simulink model "GolfSwingLogging"  (R2024b)
settings: Solver=VariableStepAuto  StartTime=0.0  StopTime=StopTime  MaxStep=0.001  RelTol=1e-3
PreLoadFcn:
  | cd(matlabdrive);
  | cd '2DModel';
PostLoadFcn:
  | %run SCRIPT_mdlWksGenerate.m;
  | mdlWks=get_param('GolfSwing','ModelWorkspace');
  | mdlWks.DataSource = 'MAT-File';
  | mdlWks.FileName = 'ModelInputs.mat';
  | mdlWks.reload;
model workspace: external: MAT-File ModelInputs.mat (data not in the file)
undefined symbols (not defined in the file or in its folder): GlobalGain, HipConstant, HipDampening, HipTimeGain, KillDampFinalValue, KillDampInitialValue, KillswitchFinalValue, KillswitchInitialValue, KillswitchStepTime, LElbowConstant, LElbowDampening, LElbowTimeGain, LScapConstant, LScapDampening, LScapPositionGain, LScapTimeGain, LShoulderConstant, LShoulderDampening, LShoulderTimeGain, LWristConstant, LWristDampening, LWristTimeGain, RElbowConstant, RElbowDampening, RElbowTimeGain, RScapConstant, RScapDampening, RScapPositionGain, RScapTimeGain, RShoulderConstant, RShoulderDampening, RShoulderTimeGain, RWristConstant, RWristDampening, RWristTimeGain, TorsoConstant, TorsoDampening, TorsoPositionGain, TorsoTimeGain, WristGain, X, Y, Z
libraries: nesl_utility x204, sm_lib x102, matrix_library x11, simulink_extras x2, simulink x1
(part 3 of 6)

== system GolfSwingLogging/Left Forearm MOF ==
  LW Global Position : Inport
  LE Global Position : Inport  Port=2
  LArmonLForearmFGlobalIn : Inport  Port=3
  LArmonLForearmTGlobalIn : Inport  Port=4
  LWristonLForearmFGlobalIn : Inport  Port=5
  LWristonLForearmTGlobalIn : Inport  Port=6
  LEAngularImpulseonForearm : Integrator
  LElbowonLForearmMOFGlobal : matrix_library/Cross Product
  LElbowonLForearmMOFLocal : Product  Multiplication=Matrix(*)
  LFCOM : sm_lib/Body Elements/Inertia Sensor  SensorExtent=BodyGroup  SpanWeldJoints=off  ExcludeGroundedBodies=off  MeasurementFrame=World  SenseMass=off  SenseCenterOfMass=on  SenseInertiaMatrix=off  SenseCenteredInertiaMatrix=off  SensePrincipalInertiaMatrix=off  SenseRotationMatrix=off  GraphicType=None  PrincipalInertiaFrameSize=20  GraphicVisPropType=SimpleVisualProperties  GraphicDiffuseColor=[0.5 0.5 0.5]  GraphicOpacity=1  GraphicSpecularColor=[0.5 0.5 0.5 1.0]  GraphicAmbientColor=[0.15 0.15 0.15 1.0]  GraphicEmissiveColor=[0.0 0.0 0.0 1.0]  GraphicShininess=75
  LWristonLForearmMOFGlobal : matrix_library/Cross Product
  LWristonLForearmMOFLocal : Product  Multiplication=Matrix(*)
  Left Forearm COM : nesl_utility/PS-Simulink Converter  PhysicalDomain=network_engine_domain  SubClassName=ps_output  LeftPortType=input  RightPortType=output  PseudoPeriodic=off  Frequencies=[]  VectorFormat=1-D array  Unit=inherit  AffineConversion=off
  R Vector Elbow Force on Left Forearm : Sum  Inputs=-+
  R Vector Wrist Force on Left Forearm : Sum  Inputs=-+
  RotationTransformLeftHand : nesl_utility/PS-Simulink Converter  PhysicalDomain=network_engine_domain  SubClassName=ps_output  LeftPortType=input  RightPortType=output  PseudoPeriodic=off  Frequencies=[]  VectorFormat=1-D array  Unit=inherit  AffineConversion=off
  SumofMomentsLEonLForearm : Sum
  SumofMomentsLForearmLocal : Product  Multiplication=Matrix(*)
  SumofMomentsLeftForearmGlobal : Sum  Inputs=++++
  Transform Sensor : sm_lib/Frames and Transforms/Transform Sensor  MeasurementFrame=World  RotationSequence=XYX  SenseAngle=off  SenseAxis=off  SenseQ=off  SenseR=on  SenseRotationSequence=off  SenseOmegaX=off  SenseOmegaY=off  SenseOmegaZ=off  SenseOmega=off  SenseQDot=off  SenseRDot=off  SenseRotationSequenceDot=off  SenseAlphaX=off  SenseAlphaY=off  SenseAlphaZ=off  SenseAlpha=off  SenseQDDot=off  SenseRDDot=off  SenseX=off  SenseY=off  SenseZ=off  SenseXYZ=off  SenseRad=off  SenseAzim=off  SenseDist=off  SenseInc=off  SenseXDot=off  SenseYDot=off  SenseZDot=off  SenseXYZDot=off  SenseRadDot=off  SenseAzimDot=off  SenseDistDot=off  SenseIncDot=off  SenseXDDot=off  SenseYDDot=off  SenseZDDot=off  SenseXYZDDot=off  SenseRadDDot=off  SenseAzimDDot=off  SenseDistDDot=off  SenseIncDDot=off
  World Frame : sm_lib/Frames and Transforms/World Frame
  Left Forearm : PMIOPort  Side=Left
  wires:
  Left Forearm COM/1 -> R Vector Elbow Force on Left Forearm/1, R Vector Wrist Force on Left Forearm/1  "LeftForearmCOM"
  LE Global Position/1 -> R Vector Elbow Force on Left Forearm/2
  LW Global Position/1 -> R Vector Wrist Force on Left Forearm/2
  R Vector Elbow Force on Left Forearm/1 -> LElbowonLForearmMOFGlobal/1
  LArmonLForearmFGlobalIn/1 -> LElbowonLForearmMOFGlobal/2
  R Vector Wrist Force on Left Forearm/1 -> LWristonLForearmMOFGlobal/1
  LWristonLForearmTGlobalIn/1 -> SumofMomentsLeftForearmGlobal/4
  LWristonLForearmFGlobalIn/1 -> LWristonLForearmMOFGlobal/2
  SumofMomentsLeftForearmGlobal/1 -> SumofMomentsLForearmLocal/2  "SumofMomentsLeftForearmGlobal"
  LWristonLForearmMOFGlobal/1 -> LWristonLForearmMOFLocal/2, SumofMomentsLeftForearmGlobal/2  "LWristonLForearmMOFGlobal"
  RotationTransformLeftHand/1 -> SumofMomentsLForearmLocal/1, LWristonLForearmMOFLocal/1, LElbowonLForearmMOFLocal/1
  LElbowonLForearmMOFGlobal/1 -> SumofMomentsLEonLForearm/2, LElbowonLForearmMOFLocal/2, SumofMomentsLeftForearmGlobal/1  "LElbowonLForearmMOFGlobal"
  SumofMomentsLEonLForearm/1 -> LEAngularImpulseonForearm/1  "SumofMomentsLEonLForearm"
  LArmonLForearmTGlobalIn/1 -> SumofMomentsLEonLForearm/1, SumofMomentsLeftForearmGlobal/3
  connections:
  LFCOM/LConn1 -- Transform Sensor/LConn1 -- Left Forearm/RConn1
  LFCOM/RConn1 -- Left Forearm COM/LConn1
  Transform Sensor/RConn1 -- World Frame/RConn1
  RotationTransformLeftHand/LConn1 -- Transform Sensor/RConn2

== system GolfSwingLogging/Left Scapula Joint ==
  note: LSOutput
  LScapForce : nesl_utility/PS-Simulink Converter  PhysicalDomain=network_engine_domain  SubClassName=ps_output  LeftPortType=input  RightPortType=output  PseudoPeriodic=off  Frequencies=[]  VectorFormat=1-D array  Unit=inherit  AffineConversion=off
  LScapPosition : nesl_utility/PS-Simulink Converter  PhysicalDomain=network_engine_domain  SubClassName=ps_output  LeftPortType=input  RightPortType=output  PseudoPeriodic=off  Frequencies=[]  VectorFormat=1-D array  Unit=inherit  AffineConversion=off
  LScapTorque1 : nesl_utility/PS-Simulink Converter  PhysicalDomain=network_engine_domain  SubClassName=ps_output  LeftPortType=input  RightPortType=output  PseudoPeriodic=off  Frequencies=[]  VectorFormat=1-D array  Unit=inherit  AffineConversion=off
  LScapVel : nesl_utility/PS-Simulink Converter  PhysicalDomain=network_engine_domain  SubClassName=ps_output  LeftPortType=input  RightPortType=output  PseudoPeriodic=off  Frequencies=[]  VectorFormat=1-D array  Unit=inherit  AffineConversion=off
  Left Scapula : sm_lib/Joints/Revolute Joint  JointMode=Normal  CompositeWrenchDir=BaseOnFollower  CompositeWrenchFrame=FollowerFrame  SenseConstraintForce=off  SenseConstraintTorque=off  SenseTotalForce=on  SenseTotalTorque=on  PositionTargetSpecify=on  PositionTargetPriority=High  PositionTargetValue=LScapStartPosition  PositionTargetValueUnits=deg  VelocityTargetSpecify=on  VelocityTargetPriority=High  VelocityTargetValue=LScapStartVelocity  VelocityTargetValueUnits=deg/s  EquilibriumPosition=0  EquilibriumPositionUnits=deg  SpringStiffness=0  SpringStiffnessUnits=N*m/deg  DampingCoefficient=0  DampingCoefficientUnits=N*m/(deg/s)  LowerLimitSpecify=off  LowerLimitBound=-90  LowerLimitBoundUnits=deg  LowerLimitStiffness=1e4  LowerLimitStiffnessUnits=N*m/deg  LowerLimitDamping=10  LowerLimitDampingUnits=N*m/(deg/s)  LowerLimitTransitionRegionWidth=0.1  LowerLimitTransitionRegionWidthUnits=deg  UpperLimitSpecify=off  UpperLimitBound=90  UpperLimitBoundUnits=deg  UpperLimitStiffness=1e4  UpperLimitStiffnessUnits=N*m/deg  UpperLimitDamping=10  UpperLimitDampingUnits=N*m/(deg/s)  UpperLimitTransitionRegionWidth=0.1  UpperLimitTransitionRegionWidthUnits=deg  TorqueActuationMode=InputTorque  MotionActuationMode=ComputedMotion  SensePosition=on  SenseVelocity=on  SenseAcceleration=off  SenseTorqueForce=off  SenseLowerLimitTorqueForce=off  SenseUpperLimitTorqueForce=off
  LSV : PMIOPort  Side=Left
  LScapTorque : PMIOPort  Port=2  Side=Left
  COM Rod Top : PMIOPort  Port=3  Side=Left
  LSP : PMIOPort  Port=4  Side=Left
  Hub : PMIOPort  Port=5  Side=Right
  connections:
  Left Scapula/LConn1 -- COM Rod Top/RConn1
  Hub/RConn1 -- Left Scapula/RConn1
  Left Scapula/LConn2 -- LScapTorque/RConn1
  LSV/RConn1 -- LScapVel/LConn1 -- Left Scapula/RConn3
  Left Scapula/RConn2 -- LScapPosition/LConn1 -- LSP/RConn1
  Left Scapula/RConn4 -- LScapForce/LConn1
  Left Scapula/RConn5 -- LScapTorque1/LConn1

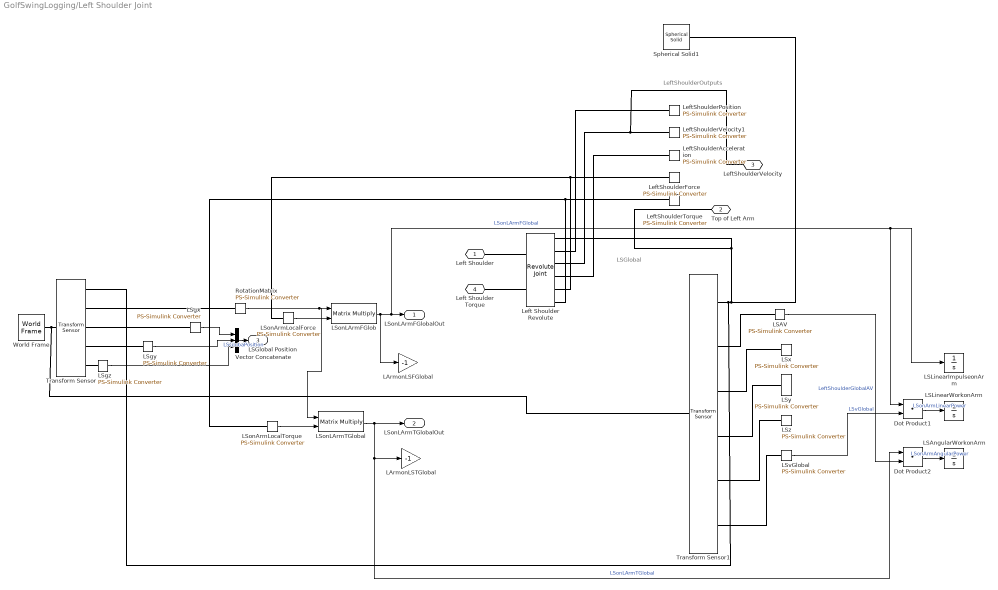
== system GolfSwingLogging/Left Shoulder Joint ==
  note: LSGlobal
  note: LeftShoulderOutputs
  Dot Product1 : DotProduct  OutDataTypeStr=Inherit: Inherit via internal rule
  Dot Product2 : DotProduct  OutDataTypeStr=Inherit: Inherit via internal rule
  LArmonLSFGlobal : Gain  Gain=-1
  LArmonLSTGlobal : Gain  Gain=-1
  LSAV : nesl_utility/PS-Simulink Converter  PhysicalDomain=network_engine_domain  SubClassName=ps_output  LeftPortType=input  RightPortType=output  PseudoPeriodic=off  Frequencies=[]  VectorFormat=1-D array  Unit=inherit  AffineConversion=off
  LSAngularWorkonArm : Integrator
  LSLinearImpulseonArm : Integrator
  LSLinearWorkonArm : Integrator
  LSgx : nesl_utility/PS-Simulink Converter  PhysicalDomain=network_engine_domain  SubClassName=ps_output  LeftPortType=input  RightPortType=output  PseudoPeriodic=off  Frequencies=[]  VectorFormat=1-D array  Unit=inherit  AffineConversion=off
  LSgy : nesl_utility/PS-Simulink Converter  PhysicalDomain=network_engine_domain  SubClassName=ps_output  LeftPortType=input  RightPortType=output  PseudoPeriodic=off  Frequencies=[]  VectorFormat=1-D array  Unit=inherit  AffineConversion=off
  LSgz : nesl_utility/PS-Simulink Converter  PhysicalDomain=network_engine_domain  SubClassName=ps_output  LeftPortType=input  RightPortType=output  PseudoPeriodic=off  Frequencies=[]  VectorFormat=1-D array  Unit=inherit  AffineConversion=off
  LSonArmLocalForce : nesl_utility/PS-Simulink Converter  PhysicalDomain=network_engine_domain  SubClassName=ps_output  LeftPortType=input  RightPortType=output  PseudoPeriodic=off  Frequencies=[]  VectorFormat=1-D array  Unit=inherit  AffineConversion=off
  LSonArmLocalTorque : nesl_utility/PS-Simulink Converter  PhysicalDomain=network_engine_domain  SubClassName=ps_output  LeftPortType=input  RightPortType=output  PseudoPeriodic=off  Frequencies=[]  VectorFormat=1-D array  Unit=inherit  AffineConversion=off
  LSonLArmFGlob : Product  Multiplication=Matrix(*)
  LSonLArmTGlobal : Product  Multiplication=Matrix(*)
  LSvGlobal : nesl_utility/PS-Simulink Converter  PhysicalDomain=network_engine_domain  SubClassName=ps_output  LeftPortType=input  RightPortType=output  PseudoPeriodic=off  Frequencies=[]  VectorFormat=1-D array  Unit=inherit  AffineConversion=off
  LSx : nesl_utility/PS-Simulink Converter  PhysicalDomain=network_engine_domain  SubClassName=ps_output  LeftPortType=input  RightPortType=output  PseudoPeriodic=off  Frequencies=[]  VectorFormat=1-D array  Unit=inherit  AffineConversion=off
  LSy : nesl_utility/PS-Simulink Converter  PhysicalDomain=network_engine_domain  SubClassName=ps_output  LeftPortType=input  RightPortType=output  PseudoPeriodic=off  Frequencies=[]  VectorFormat=1-D array  Unit=inherit  AffineConversion=off
  LSz : nesl_utility/PS-Simulink Converter  PhysicalDomain=network_engine_domain  SubClassName=ps_output  LeftPortType=input  RightPortType=output  PseudoPeriodic=off  Frequencies=[]  VectorFormat=1-D array  Unit=inherit  AffineConversion=off
  Left Shoulder Revolute : sm_lib/Joints/Revolute Joint  JointMode=Normal  CompositeWrenchDir=BaseOnFollower  CompositeWrenchFrame=FollowerFrame  SenseConstraintForce=off  SenseConstraintTorque=off  SenseTotalForce=on  SenseTotalTorque=on  PositionTargetSpecify=on  PositionTargetPriority=High  PositionTargetValue=LShoulderStartPosition  PositionTargetValueUnits=deg  VelocityTargetSpecify=on  VelocityTargetPriority=High  VelocityTargetValue=LShoulderStartVelocity  VelocityTargetValueUnits=deg/s  EquilibriumPosition=0  EquilibriumPositionUnits=deg  SpringStiffness=0  SpringStiffnessUnits=N*m/deg  DampingCoefficient=0  DampingCoefficientUnits=N*m/(deg/s)  LowerLimitSpecify=off  LowerLimitBound=-90  LowerLimitBoundUnits=deg  LowerLimitStiffness=1e4  LowerLimitStiffnessUnits=N*m/deg  LowerLimitDamping=10  LowerLimitDampingUnits=N*m/(deg/s)  LowerLimitTransitionRegionWidth=0.1  LowerLimitTransitionRegionWidthUnits=deg  UpperLimitSpecify=off  UpperLimitBound=90  UpperLimitBoundUnits=deg  UpperLimitStiffness=1e4  UpperLimitStiffnessUnits=N*m/deg  UpperLimitDamping=10  UpperLimitDampingUnits=N*m/(deg/s)  UpperLimitTransitionRegionWidth=0.1  UpperLimitTransitionRegionWidthUnits=deg  TorqueActuationMode=InputTorque  MotionActuationMode=ComputedMotion  SensePosition=on  SenseVelocity=on  SenseAcceleration=on  SenseTorqueForce=off  SenseLowerLimitTorqueForce=off  SenseUpperLimitTorqueForce=off
      settings: LogSimulationData=on
  LeftShoulderAcceleration : nesl_utility/PS-Simulink Converter  PhysicalDomain=network_engine_domain  SubClassName=ps_output  LeftPortType=input  RightPortType=output  PseudoPeriodic=off  Frequencies=[]  VectorFormat=1-D array  Unit=inherit  AffineConversion=off
  LeftShoulderForce : nesl_utility/PS-Simulink Converter  PhysicalDomain=network_engine_domain  SubClassName=ps_output  LeftPortType=input  RightPortType=output  PseudoPeriodic=off  Frequencies=[]  VectorFormat=1-D array  Unit=inherit  AffineConversion=off
  LeftShoulderPosition : nesl_utility/PS-Simulink Converter  PhysicalDomain=network_engine_domain  SubClassName=ps_output  LeftPortType=input  RightPortType=output  PseudoPeriodic=off  Frequencies=[]  VectorFormat=1-D array  Unit=inherit  AffineConversion=off
  LeftShoulderTorque : nesl_utility/PS-Simulink Converter  PhysicalDomain=network_engine_domain  SubClassName=ps_output  LeftPortType=input  RightPortType=output  PseudoPeriodic=off  Frequencies=[]  VectorFormat=1-D array  Unit=inherit  AffineConversion=off
  LeftShoulderVelocity1 : nesl_utility/PS-Simulink Converter  PhysicalDomain=network_engine_domain  SubClassName=ps_output  LeftPortType=input  RightPortType=output  PseudoPeriodic=off  Frequencies=[]  VectorFormat=1-D array  Unit=inherit  AffineConversion=off
  RotationMatrix : nesl_utility/PS-Simulink Converter  PhysicalDomain=network_engine_domain  SubClassName=ps_output  LeftPortType=input  RightPortType=output  PseudoPeriodic=off  Frequencies=[]  VectorFormat=inherit  Unit=inherit  AffineConversion=off
  Spherical Solid1 : sm_lib/Body Elements/Spherical Solid  SphereRadius=1.75  SphereRadiusUnits=in  ExportEntireGeometry=off  InertiaType=CalculateFromGeometry  BasedOnType=Density  Density=0  DensityUnits=kg/m^3  Mass=1  MassUnits=kg  CenterOfMass=[0 0 0]  CenterOfMassUnits=m  MomentsOfInertia=[1 1 1]  MomentsOfInertiaUnits=kg*m^2  ProductsOfInertia=[0 0 0]  ProductsOfInertiaUnits=kg*m^2  GraphicType=FromGeometry  MarkerShape=Sphere  MarkerSize=10  GraphicVisPropType=SimpleVisualProperties  GraphicDiffuseColor=[0.2 0.2 1.0]  GraphicOpacity=1  GraphicSpecularColor=[0.5 0.5 0.5 1.0]  GraphicAmbientColor=[0.15 0.15 0.15 1.0]  GraphicEmissiveColor=[0.0 0.0 0.0 1.0]  GraphicShininess=75  DoExposeReferenceFrame=on  SerializedFrames=<Frames/>
  Transform Sensor : sm_lib/Frames and Transforms/Transform Sensor  MeasurementFrame=World  RotationSequence=XYX  SenseAngle=off  SenseAxis=off  SenseQ=off  SenseR=on  SenseRotationSequence=off  SenseOmegaX=off  SenseOmegaY=off  SenseOmegaZ=off  SenseOmega=off  SenseQDot=off  SenseRDot=off  SenseRotationSequenceDot=off  SenseAlphaX=off  SenseAlphaY=off  SenseAlphaZ=off  SenseAlpha=off  SenseQDDot=off  SenseRDDot=off  SenseX=on  SenseY=on  SenseZ=on  SenseXYZ=off  SenseRad=off  SenseAzim=off  SenseDist=off  SenseInc=off  SenseXDot=off  SenseYDot=off  SenseZDot=off  SenseXYZDot=off  SenseRadDot=off  SenseAzimDot=off  SenseDistDot=off  SenseIncDot=off  SenseXDDot=off  SenseYDDot=off  SenseZDDot=off  SenseXYZDDot=off  SenseRadDDot=off  SenseAzimDDot=off  SenseDistDDot=off  SenseIncDDot=off
  Transform Sensor1 : sm_lib/Frames and Transforms/Transform Sensor  MeasurementFrame=World  RotationSequence=XYX  SenseAngle=off  SenseAxis=off  SenseQ=off  SenseR=off  SenseRotationSequence=off  SenseOmegaX=off  SenseOmegaY=off  SenseOmegaZ=off  SenseOmega=on  SenseQDot=off  SenseRDot=off  SenseRotationSequenceDot=off  SenseAlphaX=off  SenseAlphaY=off  SenseAlphaZ=off  SenseAlpha=off  SenseQDDot=off  SenseRDDot=off  SenseX=on  SenseY=on  SenseZ=on  SenseXYZ=off  SenseRad=off  SenseAzim=off  SenseDist=off  SenseInc=off  SenseXDot=off  SenseYDot=off  SenseZDot=off  SenseXYZDot=on  SenseRadDot=off  SenseAzimDot=off  SenseDistDot=off  SenseIncDot=off  SenseXDDot=off  SenseYDDot=off  SenseZDDot=off  SenseXYZDDot=off  SenseRadDDot=off  SenseAzimDDot=off  SenseDistDDot=off  SenseIncDDot=off
  Vector Concatenate : Concatenate  NumInputs=3
  World Frame : sm_lib/Frames and Transforms/World Frame
  Left Shoulder : PMIOPort  Side=Left
  Top of Left Arm : PMIOPort  Port=2  Side=Right
  LeftShoulderVelocity : PMIOPort  Port=3  Side=Right
  Left Shoulder Torque : PMIOPort  Port=4  Side=Right
  LSonLArmFGlobalOut : Outport
  LSonLArmTGlobalOut : Outport  Port=2
  LSGlobal Position : Outport  Port=3
  wires:
  LSonLArmTGlobal/1 -> Dot Product2/1, LArmonLSTGlobal/1, LSonLArmTGlobalOut/1  "LSonLArmTGlobal"
  LSonArmLocalForce/1 -> LSonLArmFGlob/2
  LSonArmLocalTorque/1 -> LSonLArmTGlobal/2
  RotationMatrix/1 -> LSonLArmFGlob/1, LSonLArmTGlobal/1
  LSonLArmFGlob/1 -> Dot Product1/1, LSLinearImpulseonArm/1, LSonLArmFGlobalOut/1, LArmonLSFGlobal/1  "LSonLArmFGlobal"
  LSgx/1 -> Vector Concatenate/1
  LSgy/1 -> Vector Concatenate/2
  LSgz/1 -> Vector Concatenate/3
  Vector Concatenate/1 -> LSGlobal Position/1  "LSGlobaPosition"
  Dot Product1/1 -> LSLinearWorkonArm/1  "LSonArmLinearPower"
  Dot Product2/1 -> LSAngularWorkonArm/1  "LSonArmAngularPower"
  LSvGlobal/1 -> Dot Product1/2  "LSvGlobal"
  LSAV/1 -> Dot Product2/2  "LeftShoulderGlobalAV"
  connections:
  Left Shoulder Torque/RConn1 -- Left Shoulder Revolute/LConn2
  Left Shoulder Revolute/RConn1 -- Transform Sensor1/RConn1 -- Transform Sensor/RConn1 -- Spherical Solid1/RConn1 -- Top of Left Arm/RConn1
  Left Shoulder/RConn1 -- Left Shoulder Revolute/LConn1
  World Frame/RConn1 -- Transform Sensor1/LConn1 -- Transform Sensor/LConn1
  Transform Sensor/RConn5 -- LSgz/LConn1
  LSgy/LConn1 -- Transform Sensor/RConn4
  RotationMatrix/LConn1 -- Transform Sensor/RConn2
  LSgx/LConn1 -- Transform Sensor/RConn3
  Left Shoulder Revolute/RConn5 -- LeftShoulderForce/LConn1 -- LSonArmLocalForce/LConn1
  Left Shoulder Revolute/RConn3 -- LeftShoulderVelocity1/LConn1 -- LeftShoulderVelocity/RConn1
  Left Shoulder Revolute/RConn2 -- LeftShoulderPosition/LConn1
  Left Shoulder Revolute/RConn4 -- LeftShoulderAcceleration/LConn1
  Left Shoulder Revolute/RConn6 -- LeftShoulderTorque/LConn1 -- LSonArmLocalTorque/LConn1
  LSvGlobal/LConn1 -- Transform Sensor1/RConn6
  LSAV/LConn1 -- Transform Sensor1/RConn2
  Transform Sensor1/RConn3 -- LSx/LConn1
  LSy/LConn1 -- Transform Sensor1/RConn4
  LSz/LConn1 -- Transform Sensor1/RConn5

== system GolfSwingLogging/Left Upper Arm MOF ==
  LSGlobalPosition : Inport
  LEGlobalPosition : Inport  Port=2
  LSonLArmFGlobalIn : Inport  Port=3
  LSonLArmTGlobalIn : Inport  Port=4
  LForearmonLArmFGlobalIn : Inport  Port=5
  LForearmonLArmTGlobalIn : Inport  Port=6
  LElbowonLArmMOFLocal : Product  Multiplication=Matrix(*)
  LSAngularImpulseonArm : Integrator
  LShoulderonLArmMOFGlobal : matrix_library/Cross Product
  LShoulderonLArmMOFLocal : Product  Multiplication=Matrix(*)
  LUACOM : sm_lib/Body Elements/Inertia Sensor  SensorExtent=BodyGroup  SpanWeldJoints=off  ExcludeGroundedBodies=off  MeasurementFrame=World  SenseMass=off  SenseCenterOfMass=on  SenseInertiaMatrix=off  SenseCenteredInertiaMatrix=off  SensePrincipalInertiaMatrix=off  SenseRotationMatrix=off  GraphicType=None  PrincipalInertiaFrameSize=20  GraphicVisPropType=SimpleVisualProperties  GraphicDiffuseColor=[0.5 0.5 0.5]  GraphicOpacity=1  GraphicSpecularColor=[0.5 0.5 0.5 1.0]  GraphicAmbientColor=[0.15 0.15 0.15 1.0]  GraphicEmissiveColor=[0.0 0.0 0.0 1.0]  GraphicShininess=75
  Left Upper Arm COM : nesl_utility/PS-Simulink Converter  PhysicalDomain=network_engine_domain  SubClassName=ps_output  LeftPortType=input  RightPortType=output  PseudoPeriodic=off  Frequencies=[]  VectorFormat=1-D array  Unit=inherit  AffineConversion=off
  LeftElbowonLArmMOFGlobal : matrix_library/Cross Product
  R Vector Elbow Force on Left Arm : Sum  Inputs=-+
  R Vector Shoulder Force on Left Arm : Sum  Inputs=-+
  Rotation Transform Left Arm : nesl_utility/PS-Simulink Converter  PhysicalDomain=network_engine_domain  SubClassName=ps_output  LeftPortType=input  RightPortType=output  PseudoPeriodic=off  Frequencies=[]  VectorFormat=1-D array  Unit=inherit  AffineConversion=off
  SumofMomentsLArmLocal : Product  Multiplication=Matrix(*)
  SumofMomentsLSonLArm : Sum
  SumofMomentsLeftArmGlobal : Sum  Inputs=++++
  Transform Sensor : sm_lib/Frames and Transforms/Transform Sensor  MeasurementFrame=World  RotationSequence=XYX  SenseAngle=off  SenseAxis=off  SenseQ=off  SenseR=on  SenseRotationSequence=off  SenseOmegaX=off  SenseOmegaY=off  SenseOmegaZ=off  SenseOmega=off  SenseQDot=off  SenseRDot=off  SenseRotationSequenceDot=off  SenseAlphaX=off  SenseAlphaY=off  SenseAlphaZ=off  SenseAlpha=off  SenseQDDot=off  SenseRDDot=off  SenseX=off  SenseY=off  SenseZ=off  SenseXYZ=off  SenseRad=off  SenseAzim=off  SenseDist=off  SenseInc=off  SenseXDot=off  SenseYDot=off  SenseZDot=off  SenseXYZDot=off  SenseRadDot=off  SenseAzimDot=off  SenseDistDot=off  SenseIncDot=off  SenseXDDot=off  SenseYDDot=off  SenseZDDot=off  SenseXYZDDot=off  SenseRadDDot=off  SenseAzimDDot=off  SenseDistDDot=off  SenseIncDDot=off
  World Frame : sm_lib/Frames and Transforms/World Frame
  Left Upper Arm : PMIOPort  Side=Left
  wires:
  Left Upper Arm COM/1 -> R Vector Shoulder Force on Left Arm/1, R Vector Elbow Force on Left Arm/1  "LUpperArmCOM"
  LEGlobalPosition/1 -> R Vector Elbow Force on Left Arm/2
  R Vector Elbow Force on Left Arm/1 -> LeftElbowonLArmMOFGlobal/1
  R Vector Shoulder Force on Left Arm/1 -> LShoulderonLArmMOFGlobal/1
  LSGlobalPosition/1 -> R Vector Shoulder Force on Left Arm/2
  LSonLArmFGlobalIn/1 -> LShoulderonLArmMOFGlobal/2
  LForearmonLArmFGlobalIn/1 -> LeftElbowonLArmMOFGlobal/2
  LForearmonLArmTGlobalIn/1 -> SumofMomentsLeftArmGlobal/4
  LSonLArmTGlobalIn/1 -> SumofMomentsLSonLArm/1, SumofMomentsLeftArmGlobal/3
  Rotation Transform Left Arm/1 -> SumofMomentsLArmLocal/1, LElbowonLArmMOFLocal/1, LShoulderonLArmMOFLocal/1
  LShoulderonLArmMOFGlobal/1 -> SumofMomentsLeftArmGlobal/1, SumofMomentsLSonLArm/2, LShoulderonLArmMOFLocal/2  "LShoulderonLArmMOFGlobal"
  LeftElbowonLArmMOFGlobal/1 -> SumofMomentsLeftArmGlobal/2, LElbowonLArmMOFLocal/2  "LElbowonLArmMOFGlobal"
  SumofMomentsLeftArmGlobal/1 -> SumofMomentsLArmLocal/2  "SumofMomentsLeftArmGlobal"
  SumofMomentsLSonLArm/1 -> LSAngularImpulseonArm/1  "SumofMomentsLSonLArm"
  connections:
  LUACOM/LConn1 -- Transform Sensor/LConn1 -- Left Upper Arm/RConn1
  Left Upper Arm COM/LConn1 -- LUACOM/RConn1
  Transform Sensor/RConn1 -- World Frame/RConn1
  Rotation Transform Left Arm/LConn1 -- Transform Sensor/RConn2

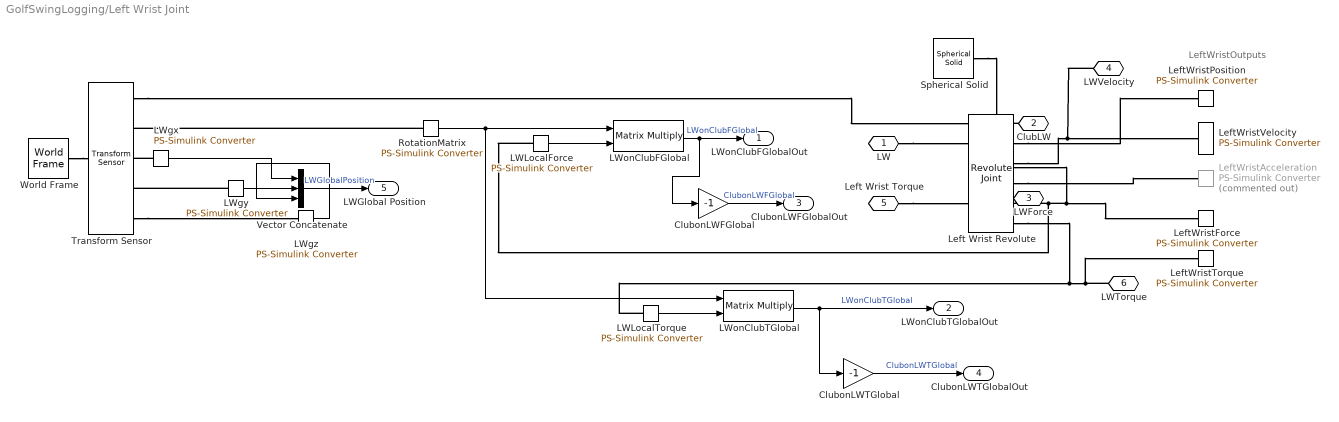
== system GolfSwingLogging/Left Wrist Joint ==
  note: LeftWristOutputs
  ClubonLWFGlobal : Gain  Gain=-1
  ClubonLWTGlobal : Gain  Gain=-1
  LWLocalForce : nesl_utility/PS-Simulink Converter  PhysicalDomain=network_engine_domain  SubClassName=ps_output  LeftPortType=input  RightPortType=output  PseudoPeriodic=off  Frequencies=[]  VectorFormat=1-D array  Unit=inherit  AffineConversion=off
  LWLocalTorque : nesl_utility/PS-Simulink Converter  PhysicalDomain=network_engine_domain  SubClassName=ps_output  LeftPortType=input  RightPortType=output  PseudoPeriodic=off  Frequencies=[]  VectorFormat=1-D array  Unit=inherit  AffineConversion=off
  LWgx : nesl_utility/PS-Simulink Converter  PhysicalDomain=network_engine_domain  SubClassName=ps_output  LeftPortType=input  RightPortType=output  PseudoPeriodic=off  Frequencies=[]  VectorFormat=1-D array  Unit=inherit  AffineConversion=off
  LWgy : nesl_utility/PS-Simulink Converter  PhysicalDomain=network_engine_domain  SubClassName=ps_output  LeftPortType=input  RightPortType=output  PseudoPeriodic=off  Frequencies=[]  VectorFormat=1-D array  Unit=inherit  AffineConversion=off
  LWgz : nesl_utility/PS-Simulink Converter  PhysicalDomain=network_engine_domain  SubClassName=ps_output  LeftPortType=input  RightPortType=output  PseudoPeriodic=off  Frequencies=[]  VectorFormat=1-D array  Unit=inherit  AffineConversion=off
  LWonClubFGlobal : Product  Multiplication=Matrix(*)
  LWonClubTGlobal : Product  Multiplication=Matrix(*)
  Left Wrist Revolute : sm_lib/Joints/Revolute Joint  JointMode=Normal  CompositeWrenchDir=BaseOnFollower  CompositeWrenchFrame=FollowerFrame  SenseConstraintForce=off  SenseConstraintTorque=off  SenseTotalForce=on  SenseTotalTorque=on  PositionTargetSpecify=on  PositionTargetPriority=High  PositionTargetValue=LWristStartPosition  PositionTargetValueUnits=deg  VelocityTargetSpecify=on  VelocityTargetPriority=High  VelocityTargetValue=LWristStartVelocity  VelocityTargetValueUnits=deg/s  EquilibriumPosition=0  EquilibriumPositionUnits=deg  SpringStiffness=0  SpringStiffnessUnits=N*m/deg  DampingCoefficient=0  DampingCoefficientUnits=N*m/(deg/s)  LowerLimitSpecify=off  LowerLimitBound=-90  LowerLimitBoundUnits=deg  LowerLimitStiffness=1e4  LowerLimitStiffnessUnits=N*m/deg  LowerLimitDamping=10  LowerLimitDampingUnits=N*m/(deg/s)  LowerLimitTransitionRegionWidth=0.1  LowerLimitTransitionRegionWidthUnits=deg  UpperLimitSpecify=off  UpperLimitBound=90  UpperLimitBoundUnits=deg  UpperLimitStiffness=1e4  UpperLimitStiffnessUnits=N*m/deg  UpperLimitDamping=10  UpperLimitDampingUnits=N*m/(deg/s)  UpperLimitTransitionRegionWidth=0.1  UpperLimitTransitionRegionWidthUnits=deg  TorqueActuationMode=InputTorque  MotionActuationMode=ComputedMotion  SensePosition=on  SenseVelocity=on  SenseAcceleration=on  SenseTorqueForce=off  SenseLowerLimitTorqueForce=off  SenseUpperLimitTorqueForce=off
      settings: LogSimulationData=on
  LeftWristAcceleration : nesl_utility/PS-Simulink Converter  Commented=on  PhysicalDomain=network_engine_domain  SubClassName=ps_output  LeftPortType=input  RightPortType=output  PseudoPeriodic=off  Frequencies=[]  VectorFormat=1-D array  Unit=inherit  AffineConversion=off
  LeftWristForce : nesl_utility/PS-Simulink Converter  PhysicalDomain=network_engine_domain  SubClassName=ps_output  LeftPortType=input  RightPortType=output  PseudoPeriodic=off  Frequencies=[]  VectorFormat=1-D array  Unit=inherit  AffineConversion=off
  LeftWristPosition : nesl_utility/PS-Simulink Converter  PhysicalDomain=network_engine_domain  SubClassName=ps_output  LeftPortType=input  RightPortType=output  PseudoPeriodic=off  Frequencies=[]  VectorFormat=1-D array  Unit=rad  AffineConversion=off
  LeftWristTorque : nesl_utility/PS-Simulink Converter  PhysicalDomain=network_engine_domain  SubClassName=ps_output  LeftPortType=input  RightPortType=output  PseudoPeriodic=off  Frequencies=[]  VectorFormat=1-D array  Unit=inherit  AffineConversion=off
  LeftWristVelocity : nesl_utility/PS-Simulink Converter  PhysicalDomain=network_engine_domain  SubClassName=ps_output  LeftPortType=input  RightPortType=output  PseudoPeriodic=off  Frequencies=[]  VectorFormat=1-D array  Unit=inherit  AffineConversion=off
  RotationMatrix : nesl_utility/PS-Simulink Converter  PhysicalDomain=network_engine_domain  SubClassName=ps_output  LeftPortType=input  RightPortType=output  PseudoPeriodic=off  Frequencies=[]  VectorFormat=1-D array  Unit=inherit  AffineConversion=off
  Spherical Solid : sm_lib/Body Elements/Spherical Solid  SphereRadius=2  SphereRadiusUnits=in  ExportEntireGeometry=off  InertiaType=CalculateFromGeometry  BasedOnType=Density  Density=0  DensityUnits=kg/m^3  Mass=1  MassUnits=kg  CenterOfMass=[0 0 0]  CenterOfMassUnits=m  MomentsOfInertia=[1 1 1]  MomentsOfInertiaUnits=kg*m^2  ProductsOfInertia=[0 0 0]  ProductsOfInertiaUnits=kg*m^2  GraphicType=FromGeometry  MarkerShape=Sphere  MarkerSize=10  GraphicVisPropType=SimpleVisualProperties  GraphicDiffuseColor=[1.0 0.8 0.4]  GraphicOpacity=1  GraphicSpecularColor=[0.5 0.5 0.5 1.0]  GraphicAmbientColor=[0.15 0.15 0.15 1.0]  GraphicEmissiveColor=[0.0 0.0 0.0 1.0]  GraphicShininess=75  DoExposeReferenceFrame=on  SerializedFrames=<Frames/>
  Transform Sensor : sm_lib/Frames and Transforms/Transform Sensor  MeasurementFrame=World  RotationSequence=XYX  SenseAngle=off  SenseAxis=off  SenseQ=off  SenseR=on  SenseRotationSequence=off  SenseOmegaX=off  SenseOmegaY=off  SenseOmegaZ=off  SenseOmega=off  SenseQDot=off  SenseRDot=off  SenseRotationSequenceDot=off  SenseAlphaX=off  SenseAlphaY=off  SenseAlphaZ=off  SenseAlpha=off  SenseQDDot=off  SenseRDDot=off  SenseX=on  SenseY=on  SenseZ=on  SenseXYZ=off  SenseRad=off  SenseAzim=off  SenseDist=off  SenseInc=off  SenseXDot=off  SenseYDot=off  SenseZDot=off  SenseXYZDot=off  SenseRadDot=off  SenseAzimDot=off  SenseDistDot=off  SenseIncDot=off  SenseXDDot=off  SenseYDDot=off  SenseZDDot=off  SenseXYZDDot=off  SenseRadDDot=off  SenseAzimDDot=off  SenseDistDDot=off  SenseIncDDot=off
  Vector Concatenate : Concatenate  NumInputs=3
  World Frame : sm_lib/Frames and Transforms/World Frame
  LW : PMIOPort  Side=Left
  ClubLW : PMIOPort  Port=2  Side=Right
  LWForce : PMIOPort  Port=3  Side=Right
  LWVelocity : PMIOPort  Port=4  Side=Right
  Left Wrist Torque : PMIOPort  Port=5  Side=Right
  LWTorque : PMIOPort  Port=6  Side=Right
  LWonClubFGlobalOut : Outport
  LWonClubTGlobalOut : Outport  Port=2
  ClubonLWFGlobalOut : Outport  Port=3
  ClubonLWTGlobalOut : Outport  Port=4
  LWGlobal Position : Outport  Port=5
  wires:
  LWLocalForce/1 -> LWonClubFGlobal/2
  LWLocalTorque/1 -> LWonClubTGlobal/2
  RotationMatrix/1 -> LWonClubFGlobal/1, LWonClubTGlobal/1
  LWonClubTGlobal/1 -> ClubonLWTGlobal/1, LWonClubTGlobalOut/1  "LWonClubTGlobal"
  ClubonLWTGlobal/1 -> ClubonLWTGlobalOut/1  "ClubonLWTGlobal"
  LWonClubFGlobal/1 -> ClubonLWFGlobal/1, LWonClubFGlobalOut/1  "LWonClubFGlobal"
  ClubonLWFGlobal/1 -> ClubonLWFGlobalOut/1  "ClubonLWFGlobal"
  LWgx/1 -> Vector Concatenate/1
  LWgz/1 -> Vector Concatenate/3
  Vector Concatenate/1 -> LWGlobal Position/1  "LWGlobalPosition"
  LWgy/1 -> Vector Concatenate/2
  connections:
  LW/RConn1 -- Left Wrist Revolute/LConn1
  Left Wrist Torque/RConn1 -- Left Wrist Revolute/LConn2
  ClubLW/RConn1 -- Transform Sensor/RConn1 -- Spherical Solid/RConn1 -- Left Wrist Revolute/RConn1
  World Frame/RConn1 -- Transform Sensor/LConn1
  RotationMatrix/LConn1 -- Transform Sensor/RConn2
  LWgx/LConn1 -- Transform Sensor/RConn3
  LWgy/LConn1 -- Transform Sensor/RConn4
  Transform Sensor/RConn5 -- LWgz/LConn1
  Left Wrist Revolute/RConn3 -- LeftWristVelocity/LConn1 -- LWVelocity/RConn1
  Left Wrist Revolute/RConn4 -- LeftWristAcceleration/LConn1
  Left Wrist Revolute/RConn2 -- LeftWristPosition/LConn1
  LWForce/RConn1 -- Left Wrist Revolute/RConn5 -- LWLocalForce/LConn1 -- LeftWristForce/LConn1
  Left Wrist Revolute/RConn6 -- LWTorque/RConn1 -- LeftWristTorque/LConn1 -- LWLocalTorque/LConn1

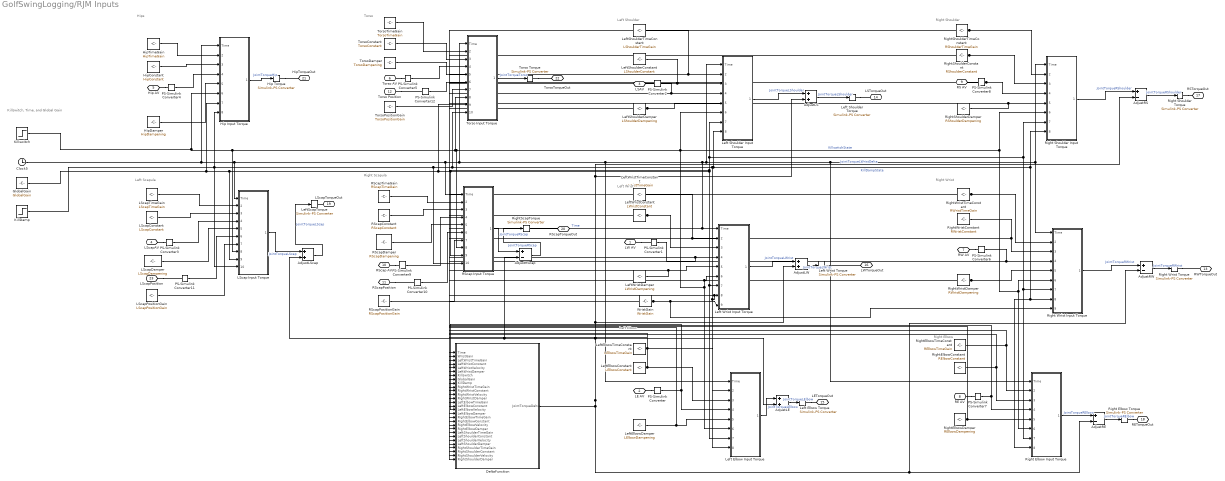
== system GolfSwingLogging/RJM Inputs ==
  note: Killswitch, Time, and Global Gain
  note: Right Scapula
  note: Left Scapula
  note: Left Shoulder
  note: Right Shoulder
  note: Right Elbow
  note: Left Elbow
  note: Torso
  note: Hips
  note: Right Wrist
  note: Left Wrist
  AdjustLE : Sum
  AdjustLS : Sum
  AdjustLScap : Sum
  AdjustLW : Sum
  AdjustRE : Sum  Inputs=+-
  AdjustRS : Sum  Inputs=+-
  AdjustRScap : Sum  Inputs=+-
  AdjustRW : Sum  Inputs=+-
  Clock5 : Clock
  DeltaFunction : MATLAB Function  TreatAsAtomicUnit=on
  GlobalGain : Constant  Value=GlobalGain
  Hip Input Torque : MATLAB Function  TreatAsAtomicUnit=on
  Hip Torque : nesl_utility/Simulink-PS Converter  PhysicalDomain=network_engine_domain  SubClassName=ps_input  LeftPortType=input  RightPortType=output  PseudoPeriodic=off  Frequencies=[]  NoiseDistribution=none  NoiseParameters=[]  Unit=N*m  AffineConversion=off  FilteringAndDerivatives=provide  SimscapeFilterOrder=1  InputFilterTimeConstant=0.001  UdotUserProvided=0
  HipConstant : Constant  Value=HipConstant
  HipDamper : Constant  Value=HipDampening
  HipTimeGain : Constant  Value=HipTimeGain
  KillDamp : Step  Time=KillswitchStepTime  Before=KillDampInitialValue  After=KillDampFinalValue  SampleTime=0
  Killswitch : Step  Time=KillswitchStepTime  Before=KillswitchInitialValue  After=KillswitchFinalValue  SampleTime=0
  LScap Input Torque : MATLAB Function  TreatAsAtomicUnit=on
  LScapConstant : Constant  Value=LScapConstant
  LScapDamper : Constant  Value=LScapDampening
  LScapPositionGain : Constant  Value=LScapPositionGain
  LScapTimeGain : Constant  Value=LScapTimeGain
  Left Elbow Input Torque : MATLAB Function  TreatAsAtomicUnit=on
  Left Elbow Torque : nesl_utility/Simulink-PS Converter  PhysicalDomain=network_engine_domain  SubClassName=ps_input  LeftPortType=input  RightPortType=output  PseudoPeriodic=off  Frequencies=[]  NoiseDistribution=none  NoiseParameters=[]  Unit=N*m  AffineConversion=off  FilteringAndDerivatives=provide  SimscapeFilterOrder=1  InputFilterTimeConstant=0.001  UdotUserProvided=0
  Left Shoulder Input Torque : MATLAB Function  TreatAsAtomicUnit=on
  Left Shoulder Torque : nesl_utility/Simulink-PS Converter  PhysicalDomain=network_engine_domain  SubClassName=ps_input  LeftPortType=input  RightPortType=output  PseudoPeriodic=off  Frequencies=[]  NoiseDistribution=none  NoiseParameters=[]  Unit=N*m  AffineConversion=off  FilteringAndDerivatives=provide  SimscapeFilterOrder=1  InputFilterTimeConstant=0.001  UdotUserProvided=0
  Left Wrist Input Torque : MATLAB Function  TreatAsAtomicUnit=on
  Left Wrist Torque : nesl_utility/Simulink-PS Converter  PhysicalDomain=network_engine_domain  SubClassName=ps_input  LeftPortType=input  RightPortType=output  PseudoPeriodic=off  Frequencies=[]  NoiseDistribution=none  NoiseParameters=[]  Unit=N*m  AffineConversion=off  FilteringAndDerivatives=provide  SimscapeFilterOrder=1  InputFilterTimeConstant=0.001  UdotUserProvided=0
  LeftElbowConstant : Constant  Value=LElbowConstant
  LeftElbowDamper : Constant  Value=LElbowDampening
  LeftElbowTimeConstant : Constant  Value=LElbowTimeGain
  LeftScapTorque : nesl_utility/Simulink-PS Converter  PhysicalDomain=network_engine_domain  SubClassName=ps_input  LeftPortType=input  RightPortType=output  PseudoPeriodic=off  Frequencies=[]  NoiseDistribution=none  NoiseParameters=[]  Unit=N*m  AffineConversion=off  FilteringAndDerivatives=provide  SimscapeFilterOrder=1  InputFilterTimeConstant=0.001  UdotUserProvided=0
  LeftShoulderConstant : Constant  Value=LShoulderConstant
  LeftShoulderDamper : Constant  Value=LShoulderDampening
  LeftShoulderTimeConstant : Constant  Value=LShoulderTimeGain
  LeftWristConstant : Constant  Value=LWristConstant
  LeftWristDamper : Constant  Value=LWristDampening
  LeftWristTimeConstant : Constant  Value=LWristTimeGain
  PS-Simulink Converter{,1..9} (10 alike) : nesl_utility/PS-Simulink Converter  PhysicalDomain=network_engine_domain  SubClassName=ps_output  LeftPortType=input  RightPortType=output  PseudoPeriodic=off  Frequencies=[]  VectorFormat=1-D array  Unit=inherit  AffineConversion=off
  PS-Simulink Converter10 : nesl_utility/PS-Simulink Converter  PhysicalDomain=network_engine_domain  SubClassName=ps_output  LeftPortType=input  RightPortType=output  PseudoPeriodic=off  Frequencies=[]  VectorFormat=inherit  Unit=inherit  AffineConversion=off
  PS-Simulink Converter11 : nesl_utility/PS-Simulink Converter  PhysicalDomain=network_engine_domain  SubClassName=ps_output  LeftPortType=input  RightPortType=output  PseudoPeriodic=off  Frequencies=[]  VectorFormat=inherit  Unit=inherit  AffineConversion=off
  PS-Simulink Converter12 : nesl_utility/PS-Simulink Converter  PhysicalDomain=network_engine_domain  SubClassName=ps_output  LeftPortType=input  RightPortType=output  PseudoPeriodic=off  Frequencies=[]  VectorFormat=inherit  Unit=inherit  AffineConversion=off
  RScap Input Torque : MATLAB Function  TreatAsAtomicUnit=on
  RScapConstant : Constant  Value=RScapConstant
  RScapDamper : Constant  Value=RScapDampening
  RScapPositionGain : Constant  Value=RScapPositionGain
  RScapTimeGain : Constant  Value=RScapTimeGain
  Right Elbow Input Torque : MATLAB Function  TreatAsAtomicUnit=on
  Right Elbow Torque : nesl_utility/Simulink-PS Converter  PhysicalDomain=network_engine_domain  SubClassName=ps_input  LeftPortType=input  RightPortType=output  PseudoPeriodic=off  Frequencies=[]  NoiseDistribution=none  NoiseParameters=[]  Unit=N*m  AffineConversion=off  FilteringAndDerivatives=provide  SimscapeFilterOrder=1  InputFilterTimeConstant=0.001  UdotUserProvided=0
  Right Shoulder Input Torque : MATLAB Function  TreatAsAtomicUnit=on
  Right Shoulder Torque : nesl_utility/Simulink-PS Converter  PhysicalDomain=network_engine_domain  SubClassName=ps_input  LeftPortType=input  RightPortType=output  PseudoPeriodic=off  Frequencies=[]  NoiseDistribution=none  NoiseParameters=[]  Unit=N*m  AffineConversion=off  FilteringAndDerivatives=provide  SimscapeFilterOrder=1  InputFilterTimeConstant=0.001  UdotUserProvided=0
  Right Wrist Input Torque : MATLAB Function  TreatAsAtomicUnit=on
  Right Wrist Torque : nesl_utility/Simulink-PS Converter  PhysicalDomain=network_engine_domain  SubClassName=ps_input  LeftPortType=input  RightPortType=output  PseudoPeriodic=off  Frequencies=[]  NoiseDistribution=none  NoiseParameters=[]  Unit=N*m  AffineConversion=off  FilteringAndDerivatives=provide  SimscapeFilterOrder=1  InputFilterTimeConstant=0.001  UdotUserProvided=0
  RightElbowConstant : Constant  Value=RElbowConstant
  RightElbowDamper : Constant  Value=RElbowDampening
  RightElbowTimeConstant : Constant  Value=RElbowTimeGain
  RightScapTorque : nesl_utility/Simulink-PS Converter  PhysicalDomain=network_engine_domain  SubClassName=ps_input  LeftPortType=input  RightPortType=output  PseudoPeriodic=off  Frequencies=[]  NoiseDistribution=none  NoiseParameters=[]  Unit=N*m  AffineConversion=off  FilteringAndDerivatives=provide  SimscapeFilterOrder=1  InputFilterTimeConstant=0.001  UdotUserProvided=0
  RightShoulderConstant : Constant  Value=RShoulderConstant
  RightShoulderDamper : Constant  Value=RShoulderDampening
  RightShoulderTimeConstant : Constant  Value=RShoulderTimeGain
  RightWristConstant : Constant  Value=RWristConstant
  RightWristDamper : Constant  Value=RWristDampening
  RightWristTimeConstant : Constant  Value=RWristTimeGain
  Torso Input Torque : MATLAB Function  TreatAsAtomicUnit=on
  Torso Torque : nesl_utility/Simulink-PS Converter  PhysicalDomain=network_engine_domain  SubClassName=ps_input  LeftPortType=input  RightPortType=output  PseudoPeriodic=off  Frequencies=[]  NoiseDistribution=none  NoiseParameters=[]  Unit=N*m  AffineConversion=off  FilteringAndDerivatives=provide  SimscapeFilterOrder=1  InputFilterTimeConstant=0.001  UdotUserProvided=0
  TorsoConstant : Constant  Value=TorsoConstant
  TorsoDamper : Constant  Value=TorsoDampening
  TorsoPositionGain : Constant  Value=TorsoPositionGain
  TorsoTimeGain : Constant  Value=TorsoTimeGain
  WristGain : Constant  Value=WristGain
  LW AV : PMIOPort  Side=Left
  LE AV : PMIOPort  Port=2  Side=Left
  LSAV : PMIOPort  Port=3  Side=Left
  LScapAV : PMIOPort  Port=4  Side=Left
  Hip AV : PMIOPort  Port=5  Side=Left
  Torso AV : PMIOPort  Port=6  Side=Left
  RW AV : PMIOPort  Port=7  Side=Left
  RE AV : PMIOPort  Port=8  Side=Left
  RS AV : PMIOPort  Port=9  Side=Left
  RScap AV : PMIOPort  Port=10  Side=Left
  RScapPosition : PMIOPort  Port=11  Side=Left
  Torso Position : PMIOPort  Port=12  Side=Left
  RWTorqueOut : PMIOPort  Port=13  Side=Right
  LSTorqueOut : PMIOPort  Port=14  Side=Right
  LETorqueOut : PMIOPort  Port=15  Side=Right
  LWTorqueOut : PMIOPort  Port=16  Side=Right
  RSTorqueOut : PMIOPort  Port=17  Side=Right
  RETorqueOut : PMIOPort  Port=18  Side=Right
  LScapTorqueOut : PMIOPort  Port=19  Side=Right
  RScapTorqueOut : PMIOPort  Port=20  Side=Right
  HipTorqueOut : PMIOPort  Port=21  Side=Right
  TorsoTorqueOut : PMIOPort  Port=22  Side=Right
  LScapPosition : PMIOPort  Port=23  Side=Right
  wires:
  GlobalGain/1 -> Torso Input Torque/9(GlobalGain), DeltaFunction/8(GlobalGain), Left Shoulder Input Torque/7(GlobalGain), Right Elbow Input Torque/7(GlobalGain), Right Wrist Input Torque/7(GlobalGain), Right Shoulder Input Torque/7(GlobalGain), Left Elbow Input Torque/7(GlobalGain), Left Wrist Input Torque/7(GlobalGain), RScap Input Torque/9(GlobalGain), LScap Input Torque/9(GlobalGain), Hip Input Torque/7(GlobalGain)
  RightElbowConstant/1 -> Right Elbow Input Torque/3(RightElbowConstant), DeltaFunction/19(RightElbowConstant)
  TorsoConstant/1 -> Torso Input Torque/3(TorsoConstant)
  TorsoTimeGain/1 -> Torso Input Torque/2(TorsoTimeGain)
  RightWristConstant/1 -> Right Wrist Input Torque/3(RightWristConstant), DeltaFunction/11(RightWristConstant)
  RightWristTimeConstant/1 -> Right Wrist Input Torque/2(RightWristTimeGain), DeltaFunction/10(RightWristTimeGain)
  RightShoulderConstant/1 -> Right Shoulder Input Torque/3(RightShoulderConstant), DeltaFunction/27(RightShoulderConstant)
  RightShoulderTimeConstant/1 -> Right Shoulder Input Torque/2(RightShoulderTimeGain), DeltaFunction/26(RightShoulderTimeGain)
  RScapConstant/1 -> RScap Input Torque/3(RScapConstant)
  RScapTimeGain/1 -> RScap Input Torque/2(RScapTimeGain)
  HipConstant/1 -> Hip Input Torque/3(HipConstant)
  HipTimeGain/1 -> Hip Input Torque/2(HipTimeGain)
  LeftWristConstant/1 -> Left Wrist Input Torque/3(LeftWristConstant), DeltaFunction/4(LeftWristConstant)
  LeftElbowConstant/1 -> Left Elbow Input Torque/3(LeftElbowConstant), DeltaFunction/15(LeftElbowConstant)
  LeftElbowTimeConstant/1 -> Left Elbow Input Torque/2(LeftElbowTimeGain), DeltaFunction/14(LeftElbowTimeGain)
  LeftShoulderTimeConstant/1 -> DeltaFunction/22(LeftShoulderTimeGain), Left Shoulder Input Torque/2(LeftShoulderTimeGain)
  LeftShoulderConstant/1 -> DeltaFunction/23(LeftShoulderConstant), Left Shoulder Input Torque/3(LeftShoulderConstant)
  LScapTimeGain/1 -> LScap Input Torque/2(LScapTimeGain)
  LScapConstant/1 -> LScap Input Torque/3(LScapConstant)
  TorsoDamper/1 -> Torso Input Torque/5(TorsoDamper)
  HipDamper/1 -> Hip Input Torque/5(HipDamper)
  RightWristDamper/1 -> Right Wrist Input Torque/5(RightWristDamper), DeltaFunction/13(RightWristDamper)
  RightElbowDamper/1 -> Right Elbow Input Torque/5(RightElbowDamper), DeltaFunction/21(RightElbowDamper)
  RightShoulderDamper/1 -> DeltaFunction/29(RightShoulderDamper), Right Shoulder Input Torque/5(RightShoulderDamper)
  RScapDamper/1 -> RScap Input Torque/5(RScapDamper)
  LeftShoulderDamper/1 -> Left Shoulder Input Torque/5(LeftShoulderDamper), DeltaFunction/25(LeftShoulderDamper)
  LScapDamper/1 -> LScap Input Torque/5(LScapDamper)
  LeftElbowDamper/1 -> Left Elbow Input Torque/5(LeftElbowDamper), DeltaFunction/17(LeftElbowDamper)
  LeftWristDamper/1 -> Left Wrist Input Torque/5(LeftWristDamper), DeltaFunction/6(LeftWristDamper)
  PS-Simulink Converter/1 -> Left Elbow Input Torque/4(LeftElbowVelocity), DeltaFunction/16(LeftElbowVelocity)
  PS-Simulink Converter9/1 -> RScap Input Torque/4(RScapVelocity)
  PS-Simulink Converter8/1 -> Right Shoulder Input Torque/4(RightShoulderVelocity), DeltaFunction/28(RightShoulderVelocity)
  PS-Simulink Converter7/1 -> Right Elbow Input Torque/4(RightElbowVelocity), DeltaFunction/20(RightElbowVelocity)
  PS-Simulink Converter6/1 -> DeltaFunction/12(RightWristVelocity), Right Wrist Input Torque/4(RightWristVelocity)
  PS-Simulink Converter5/1 -> Torso Input Torque/4(TorsoVelocity)
  PS-Simulink Converter4/1 -> Hip Input Torque/4(HipVelocity)
  PS-Simulink Converter1/1 -> Left Wrist Input Torque/4(LeftWristVelocity), DeltaFunction/5(LeftWristVelocity)
  PS-Simulink Converter2/1 -> DeltaFunction/24(LeftShoulderVelocity), Left Shoulder Input Torque/4(LeftShoulderVelocity)
  PS-Simulink Converter3/1 -> LScap Input Torque/4(LScapVelocity)
  LScapPositionGain/1 -> LScap Input Torque/7(LScapPositionGain)
  PS-Simulink Converter11/1 -> LScap Input Torque/6(LScapPosition)
  PS-Simulink Converter10/1 -> RScap Input Torque/6(RScapPosition)
  RScapPositionGain/1 -> RScap Input Torque/7(RScapPositionGain)
  TorsoPositionGain/1 -> Torso Input Torque/7(TorsoPositionGain)
  PS-Simulink Converter12/1 -> Torso Input Torque/6(TorsoPosition)
  Hip Input Torque/1(JointTorqueHips) -> Hip Torque/1  "JointTorqueHip"
  Torso Input Torque/1(JointTorqueTorso) -> Torso Torque/1  "JointTorqueTorso"
  Clock5/1 -> Right Wrist Input Torque/1(Time), Right Shoulder Input Torque/1(Time), Right Elbow Input Torque/1(Time), Left Shoulder Input Torque/1(Time), DeltaFunction/1(Time), Left Wrist Input Torque/1(Time), Left Elbow Input Torque/1(Time), Torso Input Torque/1(Time), RScap Input Torque/1(Time), LScap Input Torque/1(Time), Hip Input Torque/1(Time)  "Time"
  Killswitch/1 -> Left Elbow Input Torque/6(Killswitch), Left Wrist Input Torque/6(Killswitch), DeltaFunction/7(Killswitch), Right Wrist Input Torque/6(Killswitch), Right Elbow Input Torque/6(Killswitch), Right Shoulder Input Torque/6(Killswitch), Left Shoulder Input Torque/6(Killswitch), RScap Input Torque/8(Killswitch), Torso Input Torque/8(Killswitch), LScap Input Torque/8(Killswitch), Hip Input Torque/6(Killswitch)  "KillswitchState"
  KillDamp/1 -> Right Elbow Input Torque/8(KillDamp), Right Wrist Input Torque/8(KillDamp), Right Shoulder Input Torque/8(KillDamp), Left Shoulder Input Torque/8(KillDamp), Left Elbow Input Torque/8(KillDamp), DeltaFunction/9(KillDamp), Left Wrist Input Torque/8(KillDamp), Torso Input Torque/10(KillDamp), RScap Input Torque/10(KillDamp), Hip Input Torque/8(KillDamp), LScap Input Torque/10(KillDamp)  "KillDampState"
  Left Elbow Input Torque/1(JointTorqueLElbow) -> AdjustLE/1  "JointTorqueLElbow"
  AdjustLE/1 -> Left Elbow Torque/1  "JointTorqueLElbow"
  AdjustLS/1 -> Left Shoulder Torque/1  "JointTorqueLShoulder"
  AdjustLScap/1 -> LeftScapTorque/1  "JointTorqueLScap"
  LScap Input Torque/1(JointTorqueLScap) -> AdjustLScap/1  "JointTorqueLScap"
  AdjustRScap/1 -> RightScapTorque/1  "JointTorqueRScap"
  AdjustRS/1 -> Right Shoulder Torque/1  "JointTorqueRShoulder"
  AdjustRE/1 -> Right Elbow Torque/1  "JointTorqueRElbow"
  Right Elbow Input Torque/1(JointTorqueRElbow) -> AdjustRE/1  "JointTorqueRElbow"
  RScap Input Torque/1(JointTorqueRScap) -> AdjustRScap/1  "JointTorqueRScap"
  AdjustRW/1 -> Right Wrist Torque/1  "JointTorqueRWrist"
  Right Shoulder Input Torque/1(JointTorqueRShoulder) -> AdjustRS/1  "JointTorqueRShoulder"
  Left Shoulder Input Torque/1(JointTorqueLShoulder) -> AdjustLS/1  "JointTorqueLShoulder"
  AdjustLW/1 -> Left Wrist Torque/1  "JointTorqueLWrist"
  Left Wrist Input Torque/1(JointTorqueLWrist) -> AdjustLW/1  "JointTorqueLWrist"
  Right Wrist Input Torque/1(JointTorqueRWrist) -> AdjustRW/1  "JointTorqueRWrist"
  LeftWristTimeConstant/1 -> Left Wrist Input Torque/2(LeftWristTimeGain), DeltaFunction/3(LeftWristTimeGain)
  DeltaFunction/1(JointTorqueDelta) -> AdjustLScap/2, AdjustRScap/2, AdjustLE/2, AdjustRS/2, AdjustLS/2, AdjustLW/2, AdjustRW/2, AdjustRE/2  "JointTorqueLWristDelta"
  WristGain/1 -> Right Wrist Input Torque/9(WristGain), Left Wrist Input Torque/9(WristGain), DeltaFunction/2(WristGain)
  RightElbowTimeConstant/1 -> Right Elbow Input Torque/2(RightElbowTimeGain), DeltaFunction/18(RightElbowTimeGain)
  connections:
  Torso Torque/RConn1 -- TorsoTorqueOut/RConn1
  Right Shoulder Torque/RConn1 -- RSTorqueOut/RConn1
  Left Shoulder Torque/RConn1 -- LSTorqueOut/RConn1
  Right Elbow Torque/RConn1 -- RETorqueOut/RConn1
  LeftScapTorque/RConn1 -- LScapTorqueOut/RConn1
  RightScapTorque/RConn1 -- RScapTorqueOut/RConn1
  LE AV/RConn1 -- PS-Simulink Converter/LConn1
  LW AV/RConn1 -- PS-Simulink Converter1/LConn1
  LSAV/RConn1 -- PS-Simulink Converter2/LConn1
  LScapAV/RConn1 -- PS-Simulink Converter3/LConn1
  Hip AV/RConn1 -- PS-Simulink Converter4/LConn1
  Torso AV/RConn1 -- PS-Simulink Converter5/LConn1
  RW AV/RConn1 -- PS-Simulink Converter6/LConn1
  RE AV/RConn1 -- PS-Simulink Converter7/LConn1
  RS AV/RConn1 -- PS-Simulink Converter8/LConn1
  RScap AV/RConn1 -- PS-Simulink Converter9/LConn1
  LScapPosition/RConn1 -- PS-Simulink Converter11/LConn1
  RScapPosition/RConn1 -- PS-Simulink Converter10/LConn1
  Torso Position/RConn1 -- PS-Simulink Converter12/LConn1
  Hip Torque/RConn1 -- HipTorqueOut/RConn1
  Left Elbow Torque/RConn1 -- LETorqueOut/RConn1
  Left Wrist Torque/RConn1 -- LWTorqueOut/RConn1
  Right Wrist Torque/RConn1 -- RWTorqueOut/RConn1
